simulink model "simulation_boucle_ouverte"  (Simulink 7.0)
settings: Solver=ode45  StartTime=0.0  StopTime=15  MaxStep=1e-3  RelTol=1e-3
undefined symbols (not defined in the file or in its folder): entree_bo, pertu_bo
libraries: cstblocks x1
settings Model: Creator=adminportog  LastModifiedBy=adminportog

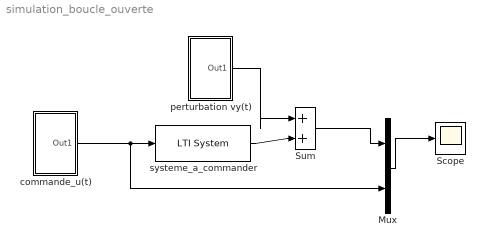
== system simulation_boucle_ouverte ==
  Mux : Mux  Inputs=2
  Scope : Scope
      settings: MaxDataPoints=50000
  Sum : Sum  Inputs=|++  OutDataType=sfix(16)  OutScaling=2^0
  commande_u(t) : Subsystem
  perturbation vy(t) : Subsystem
  systeme_a_commander : cstblocks/LTI System  SystemSampleTime=-1  sys=G1  IC=[]
  wires:
  systeme_a_commander/1 -> Sum/2
  Sum/1 -> Mux/1
  Mux/1 -> Scope/1
  commande_u(t)/1(Out1) -> systeme_a_commander/1, Mux/2
  perturbation vy(t)/1(Out1) -> Sum/1

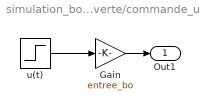
== system simulation_boucle_ouverte/commande_u(t) ==
  Gain : Gain  Gain=entree_bo  ParameterDataType=sfix(16)  ParameterScaling=2^0  OutDataType=sfix(16)  OutScaling=2^0
  u(t) : Step  Time=0  SampleTime=0
  Out1 : Outport
  wires:
  u(t)/1 -> Gain/1
  Gain/1 -> Out1/1

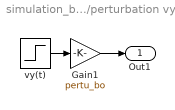
== system simulation_boucle_ouverte/perturbation vy(t) ==
  Gain1 : Gain  Gain=pertu_bo  ParameterDataType=sfix(16)  ParameterScaling=2^0  OutDataType=sfix(16)  OutScaling=2^0
  vy(t) : Step  Time=5  SampleTime=0
  Out1 : Outport
  wires:
  vy(t)/1 -> Gain1/1
  Gain1/1 -> Out1/1
